simulink model "FlOWCITSS_Mooring"  (R2019a)
settings: Solver=VariableStepAuto  StartTime=0.0  StopTime=10.0  RelTol=1e-3
values from neighbouring files (symbols this model uses):
  alphai0 = lineWeight/startingT0    (= 0.72594)    [FlOWCITSS_inputs.m]
  lineWeight = 74*9.81    (= 725.94)    [FlOWCITSS_inputs.m]
  mooringLineDepth = 400    [FlOWCITSS_inputs.m]
  mooringLineLength = 810    [FlOWCITSS_inputs.m]
  mooringLineX1 = 600    [FlOWCITSS_inputs.m]
settings Model: Creator=huffl  LastModifiedBy=huffl

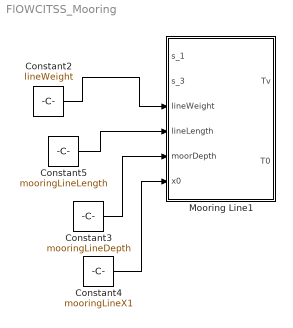
== system FlOWCITSS_Mooring ==
  Constant2 : Constant  Value=lineWeight
  Constant3 : Constant  Value=mooringLineDepth
  Constant4 : Constant  Value=mooringLineX1
  Constant5 : Constant  Value=mooringLineLength
  Mooring Line1 : Subsystem
  wires:
  Constant3/1 -> Mooring Line1/5(moorDepth)
  Constant4/1 -> Mooring Line1/6(x0)
  Constant5/1 -> Mooring Line1/4(lineLength)
  Constant2/1 -> Mooring Line1/3("lineWeight ")

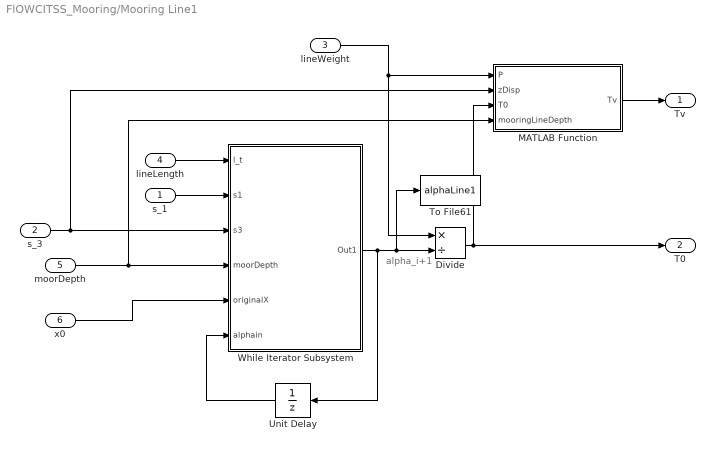
== system FlOWCITSS_Mooring/Mooring Line1 ==
  note: alpha_i+1
  "s_1 " : Inport
  "s_3 " : Inport  Port=2
  "lineWeight " : Inport  Port=3
  lineLength : Inport  Port=4
  moorDepth : Inport  Port=5
  x0 : Inport  Port=6
  Divide : Product  Inputs=*/
  MATLAB Function : MATLAB Function  TreatAsAtomicUnit=on
  To File61 : ToFile  Filename=alphaLine1  MatrixName=alphaLine1  SaveFormat=Timeseries
  Unit Delay : UnitDelay  InitialCondition=alphai0  SampleTime=-1  HasFrameUpgradeWarning=on
  While Iterator Subsystem : Subsystem  TreatAsAtomicUnit=on
  "Tv " : Outport
  "T0 " : Outport  Port=2
  wires:
  "s_1 "/1 -> While Iterator Subsystem/2(s1)
  "s_3 "/1 -> MATLAB Function/2(zDisp), While Iterator Subsystem/3("s3 ")
  Divide/1 -> MATLAB Function/3(T0), "T0 "/1
  x0/1 -> While Iterator Subsystem/5(originalX)
  MATLAB Function/1(Tv) -> "Tv "/1
  While Iterator Subsystem/1(Out1) -> To File61/1, Divide/2, Unit Delay/1
  lineLength/1 -> While Iterator Subsystem/1(l_t)
  moorDepth/1 -> While Iterator Subsystem/4(moorDepth), MATLAB Function/4(mooringLineDepth)
  "lineWeight "/1 -> MATLAB Function/1(P), Divide/1
  Unit Delay/1 -> While Iterator Subsystem/6("alphain ")

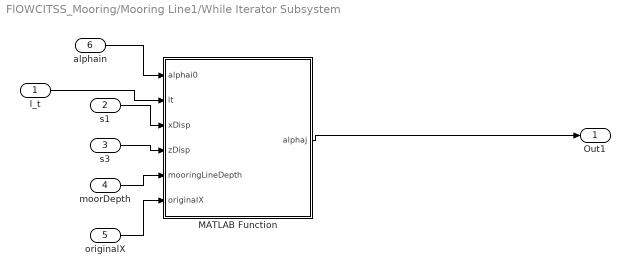
== system FlOWCITSS_Mooring/Mooring Line1/While Iterator Subsystem ==
  l_t : Inport
  s1 : Inport  Port=2
  "s3 " : Inport  Port=3
  moorDepth : Inport  Port=4
  originalX : Inport  Port=5
  "alphain " : Inport  Port=6
  MATLAB Function : MATLAB Function  TreatAsAtomicUnit=on
  Out1 : Outport
  wires:
  MATLAB Function/1(alphaj) -> Out1/1
  l_t/1 -> MATLAB Function/2(lt)
  s1/1 -> MATLAB Function/3(xDisp)
  "s3 "/1 -> MATLAB Function/4(zDisp)
  moorDepth/1 -> MATLAB Function/5(mooringLineDepth)
  originalX/1 -> MATLAB Function/6(originalX)
  "alphain "/1 -> MATLAB Function/1(alphai0)

== matlab function FlOWCITSS_Mooring/Mooring Line1/MATLAB Function ==
  data: P input; Tv output; zDisp input; T0 input; mooringLineDepth input
function Tv = fcn(P,zDisp,T0,mooringLineDepth)
h=mooringLineDepth+zDisp;
squareRoot=real(h*(h+2*(T0/P)));
Tv = P*sqrt(squareRoot);

== matlab function FlOWCITSS_Mooring/Mooring Line1/While Iterator Subsystem/MATLAB Function ==
  data: alphai0 input; alphaj output; lt input; xDisp input; zDisp input; mooringLineDepth input; originalX input
function alphaj = fcn(alphai0, lt, xDisp,zDisp,mooringLineDepth,originalX)
alphaIt=zeros(1,2000);
alphaIt(1)=[alphai0];
lprime=abs(originalX-xDisp);
h=mooringLineDepth+zDisp;
alphai=alphaIt(1);
squareRoot=real(h*(h+2/alphai));
fAlphai=sinh(alphai*(sqrt(squareRoot)+lprime-lt))-alphai*sqrt(squareRoot);
fPrimeAlphai=((h*(alphai+1)+alphai*(lprime-lt)*(sqrt(squareRoot)))*cosh(alphai*(sqrt(squareRoot)+lprime-lt)))/(alphai*sqrt(squareRoot))-(h*(alphai*h+1))/(alphai*sqrt(squareRoot));
alphaIt(2)=alphai-fAlphai/fPrimeAlphai;
count=2;
while abs(alphaIt(count)-alphaIt(count-1)) >= 0.0001
alphai=alphaIt(count);
squareRoot=real(h*(h+2/alphai));
fAlphai=sinh(alphai*(sqrt(squareRoot)+lprime-lt))-alphai*sqrt(squareRoot);
fPrimeAlphai=((h*(alphai+1)+alphai*(lprime-lt)*(sqrt(squareRoot)))*cosh(alphai*(sqrt(squareRoot)+lprime-lt)))/(alphai*sqrt(squareRoot))-(h*(alphai*h+1))/(alphai*sqrt(squareRoot));
count=count+1;
alphaIt(count)=alphai-fAlphai/fPrimeAlphai;
end
alphaj=alphaIt(count);
